simulink model "Model_symulacyjny"  (R2022a)
settings: Solver=ode3  StartTime=0.0  StopTime=600  FixedStep=1  RelTol=1e-3
values from neighbouring files (symbols this model uses):
  k = dT(end)    [Identyfikacja_nastawy.m]
  Kp = (poly_proj(2)*T - 1)/k    [Identyfikacja_nastawy.m]
  T = t(i)    [Identyfikacja_nastawy.m]
  Ti = k*Kp/wn^2/T    [Identyfikacja_nastawy.m]
  Tp = 1    [Identyfikacja_nastawy.m]
settings Model: Creator=mikos  LastModifiedBy=mikos

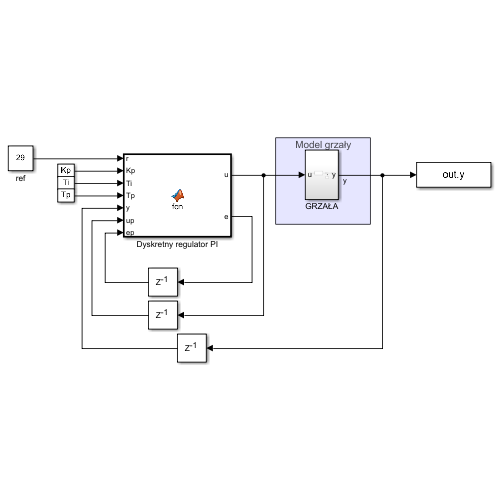
[thumbnail: Simulink's stored preview of the top-level diagram]
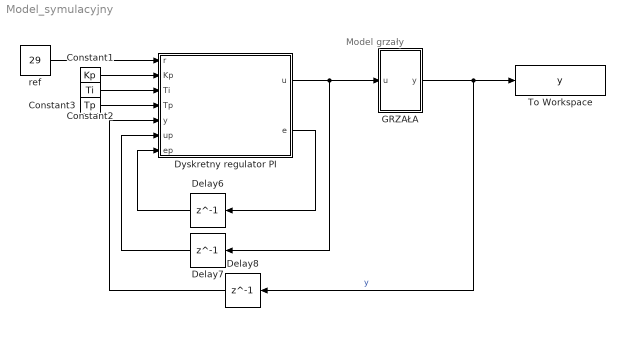
== system Model_symulacyjny ==
  note: Model grzały
  Constant1 : Constant  Value=Kp
  Constant2 : Constant  Value=Ti
  Constant3 : Constant  Value=Tp
  Delay6 : Delay  DelayLength=1
  Delay7 : Delay  DelayLength=1
  Delay8 : Delay  DelayLength=1
  Dyskretny regulator PI : MATLAB Function  TreatAsAtomicUnit=on
  GRZAŁA : Subsystem
  To Workspace : ToWorkspace  VariableName=y  SaveFormat=Timeseries  SampleTime=-1
  ref : Constant  Value=29
  wires:
  ref/1 -> Dyskretny regulator PI/1(r)
  Dyskretny regulator PI/1(u) -> Delay7/1, GRZAŁA/1(u)
  Dyskretny regulator PI/2(e) -> Delay6/1
  Delay6/1 -> Dyskretny regulator PI/7(ep)
  Delay7/1 -> Dyskretny regulator PI/6(up)
  GRZAŁA/1(y) -> Delay8/1, To Workspace/1  "y"
  Delay8/1 -> Dyskretny regulator PI/5(y)
  Constant1/1 -> Dyskretny regulator PI/2(Kp)
  Constant2/1 -> Dyskretny regulator PI/3(Ti)
  Constant3/1 -> Dyskretny regulator PI/4(Tp)

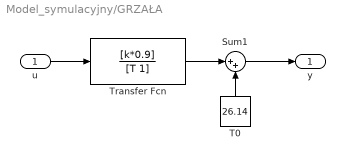
== system Model_symulacyjny/GRZAŁA ==
  u : Inport
  Sum1 : Sum  Inputs=|++
  T0 : Constant  Value=26.14
  Transfer Fcn : TransferFcn  Numerator=[k*0.9]  Denominator=[T 1]
  y : Outport
  wires:
  Transfer Fcn/1 -> Sum1/1
  u/1 -> Transfer Fcn/1
  T0/1 -> Sum1/2
  Sum1/1 -> y/1

== matlab function Model_symulacyjny/Dyskretny regulator PI ==
  data: u output; r input; Kp input; Ti input; Tp input; e output; y input; up input; ep input
function [u, e] = fcn(r, Kp, Ti, Tp, y, up, ep)

e = r - y;

uu = up + Kp*(1+Tp/Ti)*e - Kp*ep;

if uu>1
    uu = 1;
elseif uu<0
    uu = 0;
end

u = uu;
ep = e;
